simulink model "mux9bit"  (R2020a)
settings: Solver=VariableStepAuto  StartTime=0.0  StopTime=10.0  RelTol=1e-3
settings Model: Creator=kishan  LastModifiedBy=kishan

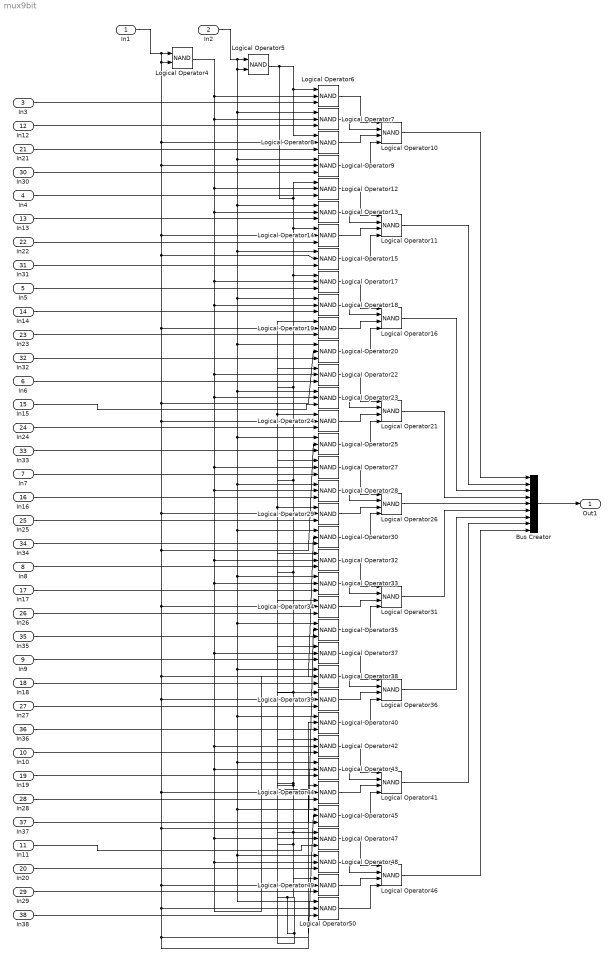
== system mux9bit ==
  In1 : Inport
  In2 : Inport  Port=2
  In3 : Inport  Port=3
  In4 : Inport  Port=4
  In5 : Inport  Port=5
  In6 : Inport  Port=6
  In7 : Inport  Port=7
  In8 : Inport  Port=8
  In9 : Inport  Port=9
  In10 : Inport  Port=10
  In11 : Inport  Port=11
  In12 : Inport  Port=12
  In13 : Inport  Port=13
  In14 : Inport  Port=14
  In15 : Inport  Port=15
  In16 : Inport  Port=16
  In17 : Inport  Port=17
  In18 : Inport  Port=18
  In19 : Inport  Port=19
  In20 : Inport  Port=20
  In21 : Inport  Port=21
  In22 : Inport  Port=22
  In23 : Inport  Port=23
  In24 : Inport  Port=24
  In25 : Inport  Port=25
  In26 : Inport  Port=26
  In27 : Inport  Port=27
  In28 : Inport  Port=28
  In29 : Inport  Port=29
  In30 : Inport  Port=30
  In31 : Inport  Port=31
  In32 : Inport  Port=32
  In33 : Inport  Port=33
  In34 : Inport  Port=34
  In35 : Inport  Port=35
  In36 : Inport  Port=36
  In37 : Inport  Port=37
  In38 : Inport  Port=38
  Bus Creator : BusCreator  Inputs=9
  Logical Operator{10..11,16,21,26,31,36,41,46} (9 alike) : Logic  Operator=NAND  Inputs=4  AllPortsSameDT=off  OutDataTypeStr=boolean
  Logical Operator{6..9,12..15,17..20,22..25,27..30,32..35,37..40,42..45,47..50} (36 alike) : Logic  Operator=NAND  Inputs=3  AllPortsSameDT=off  OutDataTypeStr=boolean
  Logical Operator4 : Logic  Operator=NAND  AllPortsSameDT=off  OutDataTypeStr=boolean
  Logical Operator5 : Logic  Operator=NAND  AllPortsSameDT=off  OutDataTypeStr=boolean
  Out1 : Outport
  wires:
  Logical Operator47/1 -> Logical Operator46/1
  Logical Operator12/1 -> Logical Operator11/1
  Logical Operator15/1 -> Logical Operator11/4
  Logical Operator21/1 -> Bus Creator/4
  In14/1 -> Logical Operator18/3
  Logical Operator6/1 -> Logical Operator10/1
  Logical Operator11/1 -> Bus Creator/2
  In3/1 -> Logical Operator6/3
  Logical Operator7/1 -> Logical Operator10/2
  Logical Operator40/1 -> Logical Operator36/4
  Logical Operator41/1 -> Bus Creator/8
  In26/1 -> Logical Operator34/3
  Logical Operator9/1 -> Logical Operator10/4
  Logical Operator36/1 -> Bus Creator/7
  Logical Operator17/1 -> Logical Operator16/1
  In2/1 -> Logical Operator50/1, Logical Operator48/1, Logical Operator45/1, Logical Operator43/1, Logical Operator40/1, Logical Operator38/1, Logical Operator35/1, Logical Operator33/1, Logical Operator30/1, Logical Operator28/1, Logical Operator25/1, Logical Operator23/1, Logical Operator20/1, Logical Operator18/1, Logical Operator15/1, Logical Operator13/1, Logical Operator9/1, Logical Operator7/1, Logical Operator5/2, Logical Operator5/1
  Logical Operator49/1 -> Logical Operator46/3
  In30/1 -> Logical Operator9/3
  In34/1 -> Logical Operator30/3
  In31/1 -> Logical Operator15/3
  In4/1 -> Logical Operator12/3
  Logical Operator10/1 -> Bus Creator/1
  Logical Operator30/1 -> Logical Operator26/4
  Logical Operator31/1 -> Bus Creator/6
  Logical Operator43/1 -> Logical Operator41/2
  In32/1 -> Logical Operator20/3
  Logical Operator44/1 -> Logical Operator41/3
  Logical Operator8/1 -> Logical Operator10/3
  Logical Operator48/1 -> Logical Operator46/2
  Logical Operator50/1 -> Logical Operator46/4
  In1/1 -> Logical Operator40/2, Logical Operator45/2, Logical Operator50/2, Logical Operator49/2, Logical Operator35/2, Logical Operator44/2, Logical Operator39/2, Logical Operator30/2, Logical Operator34/2, Logical Operator25/2, Logical Operator29/2, Logical Operator24/2, Logical Operator20/2, Logical Operator19/2, Logical Operator15/2, Logical Operator14/2, Logical Operator9/2, Logical Operator8/2, Logical Operator4/2, Logical Operator4/1
  Logical Operator26/1 -> Bus Creator/5
  Logical Operator39/1 -> Logical Operator36/3
  In18/1 -> Logical Operator38/3
  Logical Operator34/1 -> Logical Operator31/3
  Logical Operator27/1 -> Logical Operator26/1
  In25/1 -> Logical Operator29/3
  In37/1 -> Logical Operator45/3
  Logical Operator5/1 -> Logical Operator22/1, Logical Operator24/1, Logical Operator29/1, Logical Operator27/1, Logical Operator47/1, Logical Operator49/1, Logical Operator44/1, Logical Operator42/1, Logical Operator37/1, Logical Operator39/1, Logical Operator34/1, Logical Operator32/1, Logical Operator19/1, Logical Operator17/1, Logical Operator14/1, Logical Operator12/1, Logical Operator8/1, Logical Operator6/1
  Logical Operator32/1 -> Logical Operator31/1
  In17/1 -> Logical Operator33/3
  In16/1 -> Logical Operator28/3
  Logical Operator46/1 -> Bus Creator/9
  In7/1 -> Logical Operator27/3
  Logical Operator35/1 -> Logical Operator31/4
  Logical Operator28/1 -> Logical Operator26/2
  Logical Operator18/1 -> Logical Operator16/2
  In24/1 -> Logical Operator24/3
  In19/1 -> Logical Operator43/3
  In21/1 -> Logical Operator8/3
  In36/1 -> Logical Operator40/3
  Logical Operator29/1 -> Logical Operator26/3
  Logical Operator38/1 -> Logical Operator36/2
  In8/1 -> Logical Operator32/3
  In12/1 -> Logical Operator7/3
  In22/1 -> Logical Operator14/3
  In28/1 -> Logical Operator44/3
  In38/1 -> Logical Operator50/3
  In27/1 -> Logical Operator39/3
  In9/1 -> Logical Operator37/3
  Logical Operator42/1 -> Logical Operator41/1
  Logical Operator16/1 -> Bus Creator/3
  In23/1 -> Logical Operator19/3
  In6/1 -> Logical Operator22/3
  In29/1 -> Logical Operator49/3
  Logical Operator25/1 -> Logical Operator21/4
  Logical Operator24/1 -> Logical Operator21/3
  Bus Creator/1 -> Out1/1
  Logical Operator37/1 -> Logical Operator36/1
  In5/1 -> Logical Operator17/3
  Logical Operator20/1 -> Logical Operator16/4
  Logical Operator45/1 -> Logical Operator41/4
  Logical Operator4/1 -> Logical Operator38/2, Logical Operator48/2, Logical Operator47/2, Logical Operator43/2, Logical Operator42/2, Logical Operator37/2, Logical Operator33/2, Logical Operator32/2, Logical Operator28/2, Logical Operator27/2, Logical Operator23/2, Logical Operator22/2, Logical Operator18/2, Logical Operator17/2, Logical Operator13/2, Logical Operator12/2, Logical Operator7/2, Logical Operator6/2
  Logical Operator19/1 -> Logical Operator16/3
  In33/1 -> Logical Operator25/3
  In10/1 -> Logical Operator42/3
  In15/1 -> Logical Operator23/3
  In13/1 -> Logical Operator13/3
  In11/1 -> Logical Operator47/3
  In20/1 -> Logical Operator48/3
  Logical Operator23/1 -> Logical Operator21/2
  In35/1 -> Logical Operator35/3
  Logical Operator13/1 -> Logical Operator11/2
  Logical Operator22/1 -> Logical Operator21/1
  Logical Operator33/1 -> Logical Operator31/2
  Logical Operator14/1 -> Logical Operator11/3
